simulink model "gm_sampleModel1443_sub"  (R2023a)
settings: Solver=VariableStepAuto  StartTime=0.0  StopTime=10.0  RelTol=1e-3
libraries: hdlsllib x2, simulink x1
settings Model: Creator=user1  LastModifiedBy=user1
settings OptimizationCC: BlockReduction=off  ConditionallyExecuteInputs=off
settings DebuggingCC: InheritedTsInSrcMsg=none

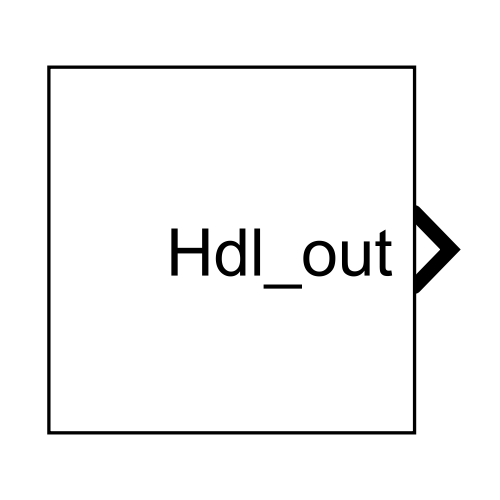
[thumbnail: Simulink's stored preview of the top-level diagram]
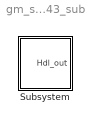
== system gm_sampleModel1443_sub ==
  Subsystem : Subsystem

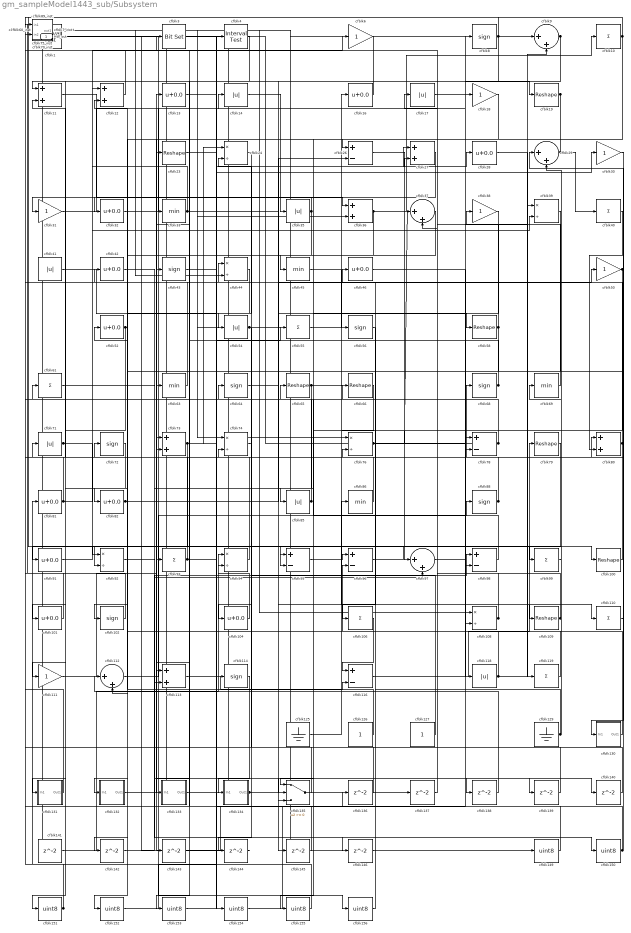
== system gm_sampleModel1443_sub/Subsystem ==
  cfblk1 : hdlsllib/Logic and Bit Operations/Interval Test  IntervalClosedRight=on  uplimit=0.5  IntervalClosedLeft=on  lowlimit=-0.5  OutDataTypeStr=uint8
  cfblk{10,40,55,61,93,99,106,110,119} (9 alike) : Sum  Inputs=+  OutDataTypeStr=uint8
  cfblk{19,23,58,65..66,79,100,109} (8 alike) : Reshape
  cfblk{13,16,28,32,42,46,52,81..82,91,101,104} (12 alike) : Bias  Bias=0.0  SaturateOnIntegerOverflow=off
  cfblk{8,43,56,64,68,72,88,102,114} (9 alike) : Signum
  cfblk103_inst : Subsystem
  cfblk{24,39,44,74,76,92,94,108} (8 alike) : Product  Inputs=*/  OutDataTypeStr=uint8  RndMeth=Zero  SaturateOnIntegerOverflow=on
  cfblk{11..12,27,36,73,80,113} (7 alike) : Sum  OutDataTypeStr=uint8
  cfblk{6,18,30..31,38,50,111} (7 alike) : Gain  OutDataTypeStr=uint8
  cfblk{9,29,37,97,112} (5 alike) : Sum  Inputs=|++  OutDataTypeStr=uint8
  cfblk115_inst : Subsystem
  cfblk{26,78,95..96,98,116} (6 alike) : Sum  Inputs=+-  OutDataTypeStr=uint8
  cfblk{14,17,35,41,54,71,85,118} (8 alike) : Abs  OutDataTypeStr=uint8  SaturateOnIntegerOverflow=off
  cfblk125 : Ground
  cfblk126 : Constant  OutDataTypeStr=uint8  SampleTime=-1
  cfblk127 : Constant  OutDataTypeStr=uint8  SampleTime=-1
  cfblk129 : Ground
  cfblk130 : Subsystem
  cfblk131 : Subsystem
  cfblk132 : Subsystem
  cfblk133 : Subsystem
  cfblk134 : Subsystem
  cfblk135 : Switch  OutDataTypeStr=uint8  SaturateOnIntegerOverflow=off  InputSameDT=off
  cfblk{136..146} (11 alike) : Delay  SampleTime=1
  cfblk{149..156} (8 alike) : DataTypeConversion  OutDataTypeStr=uint8  SaturateOnIntegerOverflow=off  RndMeth=Floor
  cfblk15_inst : Subsystem
  cfblk3 : simulink/Logic and Bit Operations/Bit Set  iBit=0
      settings: LibrarySourceBlock=|
      | hdlsllib/Logic and Bit
      | Operations/Bit Set
  cfblk{33,45,63,69,86} (5 alike) : MinMax  OutDataTypeStr=uint8
  cfblk4 : hdlsllib/Logic and Bit Operations/Interval Test  IntervalClosedRight=on  uplimit=0.5  IntervalClosedLeft=on  lowlimit=-0.5  OutDataTypeStr=uint8
  cfblk57_inst : Subsystem
  cfblk59_inst : Subsystem
  cfblk60_inst : Subsystem
  cfblk67_inst : Subsystem
  cfblk70_inst : Subsystem
  cfblk75_inst : Subsystem
  cfblk7_inst : Subsystem
  cfblk89_inst : Subsystem
  Hdl_out : Outport  OutDataTypeStr=uint8  SampleTime=1
  wires:
  cfblk1/1 -> cfblk156/1
  cfblk10/1 -> cfblk92/2, cfblk143/1
  cfblk100/1 -> cfblk68/1
  cfblk101/1 -> cfblk7_inst/1(in1)
  cfblk102/1 -> cfblk57_inst/1(in1)
  cfblk103_inst/1(out1) -> cfblk135/2
  cfblk104/1 -> cfblk94/1
  cfblk106/1 -> cfblk116/1
  cfblk108/1 -> cfblk70_inst/2(in2), cfblk64/1
  cfblk109/1 -> cfblk75_inst/2(in2), cfblk59_inst/1(in1), cfblk15_inst/2(in2)
  cfblk11/1 -> cfblk36/1
  cfblk110/1 -> cfblk29/1
  cfblk111/1 -> cfblk13/1
  cfblk112/1 -> cfblk88/1
  cfblk113/1 -> cfblk116/2
  cfblk114/1 -> cfblk134/1(In1)
  cfblk115_inst/1(out1) -> cfblk108/1
  cfblk116/1 -> cfblk79/1
  cfblk118/1 -> cfblk96/2, cfblk9/2
  cfblk119/1 -> cfblk72/1
  cfblk12/1 -> cfblk70_inst/1(in1)
  cfblk125/1 -> cfblk86/1
  cfblk126/1 -> cfblk12/2
  cfblk127/1 -> cfblk44/1
  cfblk129/1 -> cfblk46/1, cfblk29/2
  cfblk13/1 -> cfblk154/1
  cfblk130/1(Out1) -> cfblk52/1
  cfblk131/1(Out1) -> cfblk115_inst/2(in2)
  cfblk132/1(Out1) -> cfblk43/1
  cfblk133/1(Out1) -> cfblk55/1
  cfblk134/1(Out1) -> cfblk140/1, cfblk139/1
  cfblk135/1 -> cfblk93/1
  cfblk136/1 -> cfblk60_inst/1(in1)
  cfblk137/1 -> cfblk37/2
  cfblk138/1 -> cfblk112/1
  cfblk139/1 -> cfblk73/1
  cfblk14/1 -> cfblk35/1
  cfblk140/1 -> cfblk24/2
  cfblk141/1 -> cfblk94/2
  cfblk142/1 -> cfblk98/1
  cfblk143/1 -> cfblk78/1
  cfblk144/1 -> cfblk1/1
  cfblk145/1 -> cfblk89_inst/2(in2)
  cfblk146/1 -> cfblk76/2
  cfblk149/1 -> cfblk3/1
  cfblk15_inst/1(out1) -> cfblk36/2
  cfblk150/1 -> cfblk80/1, cfblk103_inst/1(in1)
  cfblk151/1 -> cfblk81/1, cfblk115_inst/1(in1)
  cfblk152/1 -> cfblk4/1
  cfblk153/1 -> cfblk136/1
  cfblk154/1 -> cfblk18/1
  cfblk155/1 -> cfblk60_inst/2(in2)
  cfblk156/1 -> cfblk66/1
  cfblk16/1 -> cfblk11/1
  cfblk17/1 -> cfblk19/1
  cfblk18/1 -> cfblk153/1
  cfblk19/1 -> cfblk95/2, cfblk152/1
  cfblk23/1 -> cfblk99/1
  cfblk24/1 -> cfblk54/1
  cfblk26/1 -> cfblk97/1
  cfblk27/1 -> cfblk91/1
  cfblk28/1 -> cfblk119/1
  cfblk29/1 -> cfblk26/1, cfblk40/1
  cfblk3/1 -> cfblk150/1
  cfblk30/1 -> cfblk130/1(In1)
  cfblk31/1 -> cfblk14/1
  cfblk32/1 -> cfblk8/1
  cfblk33/1 -> cfblk58/1, cfblk12/1
  cfblk35/1 -> cfblk32/1, cfblk113/1
  cfblk36/1 -> cfblk142/1, cfblk10/1
  cfblk37/1 -> cfblk45/1
  cfblk38/1 -> cfblk85/1
  cfblk39/1 -> cfblk135/1
  cfblk4/1 -> cfblk151/1
  cfblk40/1 -> cfblk80/2
  cfblk41/1 -> cfblk74/1
  cfblk42/1 -> cfblk146/1
  cfblk43/1 -> cfblk30/1
  cfblk44/1 -> cfblk132/1(In1)
  cfblk45/1 -> cfblk78/2
  cfblk46/1 -> cfblk118/1
  cfblk50/1 -> cfblk108/2, cfblk63/1
  cfblk52/1 -> cfblk112/2, cfblk101/1
  cfblk54/1 -> cfblk27/2, cfblk104/1, cfblk50/1
  cfblk55/1 -> cfblk16/1
  cfblk56/1 -> cfblk106/1
  cfblk57_inst/1(out1) -> cfblk56/1
  cfblk58/1 -> cfblk82/1, cfblk7_inst/2(in2), cfblk67_inst/2(in2)
  cfblk59_inst/1(out1) -> cfblk141/1
  cfblk6/1 -> cfblk31/1
  cfblk60_inst/1(out1) -> cfblk76/1
  cfblk61/1 -> cfblk138/1
  cfblk63/1 -> cfblk42/1
  cfblk64/1 -> cfblk145/1
  cfblk65/1 -> cfblk113/2, cfblk109/1
  cfblk66/1 -> cfblk155/1
  cfblk67_inst/1(out1) -> cfblk9/1
  cfblk68/1 -> cfblk17/1, cfblk33/1
  cfblk69/1 -> cfblk38/1
  cfblk7_inst/1(out1) -> cfblk137/1
  cfblk70_inst/1(out1) -> cfblk41/1
  cfblk71/1 -> cfblk92/1, cfblk39/2
  cfblk72/1 -> cfblk111/1
  cfblk73/1 -> cfblk28/1, cfblk102/1, cfblk24/1
  cfblk74/1 -> cfblk144/1
  cfblk75_inst/1(out1) -> cfblk44/2
  cfblk76/1 -> cfblk37/1, cfblk100/1
  cfblk78/1 -> cfblk89_inst/1(in1), Hdl_out/1
  cfblk79/1 -> cfblk131/1(In1)
  cfblk8/1 -> cfblk67_inst/1(in1), cfblk135/3
  cfblk80/1 -> cfblk73/2, cfblk103_inst/2(in2)
  cfblk81/1 -> cfblk15_inst/1(in1), cfblk6/1
  cfblk82/1 -> cfblk27/1, cfblk26/2, cfblk110/1
  cfblk85/1 -> cfblk57_inst/2(in2), cfblk74/2
  cfblk86/1 -> cfblk11/2
  cfblk88/1 -> cfblk71/1, cfblk59_inst/2(in2)
  cfblk89_inst/1(out1) -> cfblk149/1
  cfblk9/1 -> cfblk23/1, cfblk133/1(In1)
  cfblk91/1 -> cfblk95/1
  cfblk92/1 -> cfblk97/2
  cfblk93/1 -> cfblk114/1, cfblk61/1
  cfblk94/1 -> cfblk75_inst/1(in1)
  cfblk95/1 -> cfblk96/1
  cfblk96/1 -> cfblk98/2
  cfblk97/1 -> cfblk39/1
  cfblk98/1 -> cfblk65/1
  cfblk99/1 -> cfblk69/1

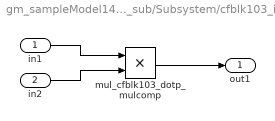
== system gm_sampleModel1443_sub/Subsystem/cfblk103_inst ==
  in1 : Inport  OutDataTypeStr=uint8  SampleTime=1
  in2 : Inport  Port=2  OutDataTypeStr=uint8  SampleTime=1
  mul_cfblk103_dotp_mulcomp : Product  Inputs=**  OutDataTypeStr=uint8  SampleTime=1
  out1 : Outport  OutDataTypeStr=uint8  SampleTime=1
  wires:
  in1/1 -> mul_cfblk103_dotp_mulcomp/1
  in2/1 -> mul_cfblk103_dotp_mulcomp/2
  mul_cfblk103_dotp_mulcomp/1 -> out1/1

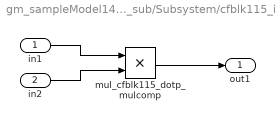
== system gm_sampleModel1443_sub/Subsystem/cfblk115_inst ==
  in1 : Inport  OutDataTypeStr=uint8  SampleTime=1
  in2 : Inport  Port=2  OutDataTypeStr=uint8  SampleTime=1
  mul_cfblk115_dotp_mulcomp : Product  Inputs=**  OutDataTypeStr=uint8  SampleTime=1
  out1 : Outport  OutDataTypeStr=uint8  SampleTime=1
  wires:
  in1/1 -> mul_cfblk115_dotp_mulcomp/1
  in2/1 -> mul_cfblk115_dotp_mulcomp/2
  mul_cfblk115_dotp_mulcomp/1 -> out1/1

== system gm_sampleModel1443_sub/Subsystem/cfblk130 ==
  In1 : Inport  OutDataTypeStr=uint8  PortDimensions=1  SampleTime=1
  Out1 : Outport  SampleTime=1
  wires:
  In1/1 -> Out1/1

== system gm_sampleModel1443_sub/Subsystem/cfblk131 ==
  In1 : Inport  OutDataTypeStr=uint8  PortDimensions=1  SampleTime=1
  Out1 : Outport  SampleTime=1
  wires:
  In1/1 -> Out1/1

== system gm_sampleModel1443_sub/Subsystem/cfblk132 ==
  In1 : Inport  OutDataTypeStr=uint8  PortDimensions=1  SampleTime=1
  Out1 : Outport  SampleTime=1
  wires:
  In1/1 -> Out1/1

== system gm_sampleModel1443_sub/Subsystem/cfblk133 ==
  In1 : Inport  OutDataTypeStr=uint8  PortDimensions=1  SampleTime=1
  Out1 : Outport  SampleTime=1
  wires:
  In1/1 -> Out1/1

== system gm_sampleModel1443_sub/Subsystem/cfblk134 ==
  In1 : Inport  OutDataTypeStr=uint8  PortDimensions=1  SampleTime=1
  Out1 : Outport  SampleTime=1
  wires:
  In1/1 -> Out1/1

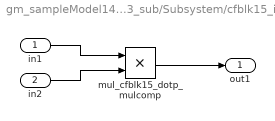
== system gm_sampleModel1443_sub/Subsystem/cfblk15_inst ==
  in1 : Inport  OutDataTypeStr=uint8  SampleTime=1
  in2 : Inport  Port=2  OutDataTypeStr=uint8  SampleTime=1
  mul_cfblk15_dotp_mulcomp : Product  Inputs=**  OutDataTypeStr=uint8  SampleTime=1
  out1 : Outport  OutDataTypeStr=uint8  SampleTime=1
  wires:
  in1/1 -> mul_cfblk15_dotp_mulcomp/1
  in2/1 -> mul_cfblk15_dotp_mulcomp/2
  mul_cfblk15_dotp_mulcomp/1 -> out1/1

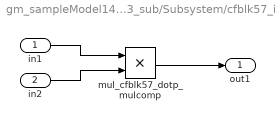
== system gm_sampleModel1443_sub/Subsystem/cfblk57_inst ==
  in1 : Inport  OutDataTypeStr=uint8  SampleTime=1
  in2 : Inport  Port=2  OutDataTypeStr=uint8  SampleTime=1
  mul_cfblk57_dotp_mulcomp : Product  Inputs=**  OutDataTypeStr=uint8  SampleTime=1
  out1 : Outport  OutDataTypeStr=uint8  SampleTime=1
  wires:
  in1/1 -> mul_cfblk57_dotp_mulcomp/1
  in2/1 -> mul_cfblk57_dotp_mulcomp/2
  mul_cfblk57_dotp_mulcomp/1 -> out1/1

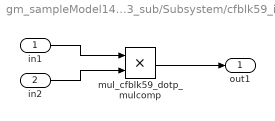
== system gm_sampleModel1443_sub/Subsystem/cfblk59_inst ==
  in1 : Inport  OutDataTypeStr=uint8  SampleTime=1
  in2 : Inport  Port=2  OutDataTypeStr=uint8  SampleTime=1
  mul_cfblk59_dotp_mulcomp : Product  Inputs=**  OutDataTypeStr=uint8  SampleTime=1
  out1 : Outport  OutDataTypeStr=uint8  SampleTime=1
  wires:
  in1/1 -> mul_cfblk59_dotp_mulcomp/1
  in2/1 -> mul_cfblk59_dotp_mulcomp/2
  mul_cfblk59_dotp_mulcomp/1 -> out1/1

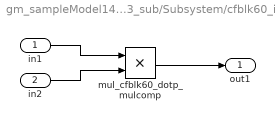
== system gm_sampleModel1443_sub/Subsystem/cfblk60_inst ==
  in1 : Inport  OutDataTypeStr=uint8  SampleTime=1
  in2 : Inport  Port=2  OutDataTypeStr=uint8  SampleTime=1
  mul_cfblk60_dotp_mulcomp : Product  Inputs=**  OutDataTypeStr=uint8  SampleTime=1
  out1 : Outport  OutDataTypeStr=uint8  SampleTime=1
  wires:
  in1/1 -> mul_cfblk60_dotp_mulcomp/1
  in2/1 -> mul_cfblk60_dotp_mulcomp/2
  mul_cfblk60_dotp_mulcomp/1 -> out1/1

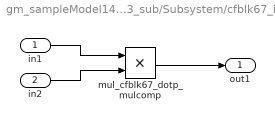
== system gm_sampleModel1443_sub/Subsystem/cfblk67_inst ==
  in1 : Inport  OutDataTypeStr=uint8  SampleTime=1
  in2 : Inport  Port=2  OutDataTypeStr=uint8  SampleTime=1
  mul_cfblk67_dotp_mulcomp : Product  Inputs=**  OutDataTypeStr=uint8  SampleTime=1
  out1 : Outport  OutDataTypeStr=uint8  SampleTime=1
  wires:
  in1/1 -> mul_cfblk67_dotp_mulcomp/1
  in2/1 -> mul_cfblk67_dotp_mulcomp/2
  mul_cfblk67_dotp_mulcomp/1 -> out1/1

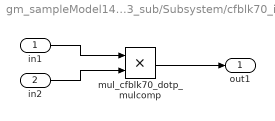
== system gm_sampleModel1443_sub/Subsystem/cfblk70_inst ==
  in1 : Inport  OutDataTypeStr=uint8  SampleTime=1
  in2 : Inport  Port=2  OutDataTypeStr=uint8  SampleTime=1
  mul_cfblk70_dotp_mulcomp : Product  Inputs=**  OutDataTypeStr=uint8  SampleTime=1
  out1 : Outport  OutDataTypeStr=uint8  SampleTime=1
  wires:
  in1/1 -> mul_cfblk70_dotp_mulcomp/1
  in2/1 -> mul_cfblk70_dotp_mulcomp/2
  mul_cfblk70_dotp_mulcomp/1 -> out1/1

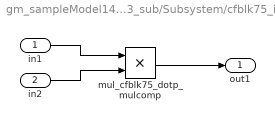
== system gm_sampleModel1443_sub/Subsystem/cfblk75_inst ==
  in1 : Inport  OutDataTypeStr=uint8  SampleTime=1
  in2 : Inport  Port=2  OutDataTypeStr=uint8  SampleTime=1
  mul_cfblk75_dotp_mulcomp : Product  Inputs=**  OutDataTypeStr=uint8  SampleTime=1
  out1 : Outport  OutDataTypeStr=uint8  SampleTime=1
  wires:
  in1/1 -> mul_cfblk75_dotp_mulcomp/1
  in2/1 -> mul_cfblk75_dotp_mulcomp/2
  mul_cfblk75_dotp_mulcomp/1 -> out1/1

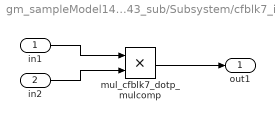
== system gm_sampleModel1443_sub/Subsystem/cfblk7_inst ==
  in1 : Inport  OutDataTypeStr=uint8  SampleTime=1
  in2 : Inport  Port=2  OutDataTypeStr=uint8  SampleTime=1
  mul_cfblk7_dotp_mulcomp : Product  Inputs=**  OutDataTypeStr=uint8  SampleTime=1
  out1 : Outport  OutDataTypeStr=uint8  SampleTime=1
  wires:
  in1/1 -> mul_cfblk7_dotp_mulcomp/1
  in2/1 -> mul_cfblk7_dotp_mulcomp/2
  mul_cfblk7_dotp_mulcomp/1 -> out1/1

== system gm_sampleModel1443_sub/Subsystem/cfblk89_inst ==
  in1 : Inport  OutDataTypeStr=uint8  SampleTime=1
  in2 : Inport  Port=2  OutDataTypeStr=uint8  SampleTime=1
  mul_cfblk89_dotp_mulcomp : Product  Inputs=**  OutDataTypeStr=uint8  SampleTime=1
  out1 : Outport  OutDataTypeStr=uint8  SampleTime=1
  wires:
  in1/1 -> mul_cfblk89_dotp_mulcomp/1
  in2/1 -> mul_cfblk89_dotp_mulcomp/2
  mul_cfblk89_dotp_mulcomp/1 -> out1/1
